simulink model "full_plant20"  (R2021a)
settings: Solver=VariableStepAuto  StartTime=0.0  StopTime=10000  RelTol=1e-3
values from neighbouring files (symbols this model uses):
  alpha_c = 0.00001    (= 1e-05)    [full_plant.m]    (also in full_plant_20.m; policy.m; reactor_core.m)
  alpha_f = -0.00005    (= -5e-05)    [full_plant.m]    (also in full_plant_20.m; policy.m; reactor_core.m)
  beta = p ^ 0.25    (= 0)    [XSteam.m]    (also in XSteam_h_ps.m; full_plant.m = sum(betas); full_plant_20.m = sum(betas); policy.m = sum(betas))
  betas = [0.000215; 0.001424; 0.001274; 0.002568; 0.000748; 0.000273]    [full_plant.m]    (also in full_plant_20.m; policy.m; reactor_core.m)
  err_weights = 0.3    [full_plant_20.m]    (also in sg.m = 0.5)
  eta = 0.85    [PIturing.m]    (also in XSteam.m = h / 3000; XSteam_h_ps.m = h / 3000; full_plant.m = 0.809489; full_plant_20.m = 0.809489)
  eta_all = Pt0 / P_thermal0    [full_plant_20.m]
  ff = 0.98    [full_plant.m]    (also in full_plant_20.m; policy.m; reactor_core.m)
  Gr = 0.0001 * beta    [full_plant_20.m]    (also in reactor_core.m = 0.00001 * beta)
  h_fw = h_sg_out0 - P_thermal0 * 1e3 / num_sg / W_o0    [full_plant.m]    (also in full_plant_20.m; policy.m = h_sg_out0 - P_thermal0 * 1e3 / num_sg / W0; reactor_core.m = h_sg_out0 - P_thermal0 * 1e3 / num_sg / W0; sg.m = h_sg_out0 - P_thermal0 * 1e3 / num_sg / W0)
  J = 8500    [PIturing.m]    (also in full_plant.m; full_plant_20.m; policy.m; reactor_core.m)
  ki_sg = 1.5    [full_plant_20.m]
  kp_sg = 1.6    [full_plant_20.m]
  Lambda = 0.0001    [full_plant.m]    (also in full_plant_20.m; policy.m; reactor_core.m)
  lambdas = [0.0124; 0.0305; 0.1110; 0.3010; 1.1400; 3.0100]    [full_plant.m]    (also in full_plant_20.m; policy.m; reactor_core.m)
  M = M_sg * 2    (= 92.7075812274)    [full_plant.m]    (also in full_plant_20.m; policy.m; reactor_core.m)
  M_sg = P_thermal0 / (T_h0 - T_c0) / num_sg    (= 46.3537906137)    [full_plant.m]    (also in full_plant_20.m; policy.m; reactor_core.m; sg.m)
  mu_c = 70.5    [full_plant.m]    (also in full_plant_20.m; policy.m; reactor_core.m)
  mu_f = 26.3    [full_plant.m]    (also in full_plant_20.m; policy.m; reactor_core.m)
  mu_m = 8.46    [full_plant.m]    (also in full_plant_20.m; policy.m; reactor_core.m; sg.m)
  mu_p = 141.0    (= 141)    [full_plant.m]    (also in full_plant_20.m; policy.m; reactor_core.m; sg.m)
  Ndes = 3600    [PIturing.m]    (also in full_plant.m; full_plant_20.m; policy.m; reactor_core.m)
  num_sg = 2    [full_plant.m]    (also in full_plant_20.m; policy.m; reactor_core.m; sg.m)
  Omega = P_thermal0 * ff / (T_f0 - T_h0)    (= 6.72125630959)    [full_plant.m]    (also in full_plant_20.m; policy.m; reactor_core.m)
  P_sg0 = 6.38    [full_plant.m]    (also in full_plant_20.m; policy.m; reactor_core.m; sg.m)
  P_thermal0 = 2568    [full_plant.m]    (also in full_plant_20.m; policy.m; reactor_core.m; sg.m)
  Pc = 0.008    [PIturing.m]    (also in full_plant.m; full_plant_20.m; policy.m; reactor_core.m)
  Pg0 = 819    [PIturing.m]    (also in full_plant.m = Pt0; full_plant_20.m = Pt0; policy.m = Pt0; reactor_core.m = Pt0)
  SG_gain = 0.002    [full_plant_20.m]
  T_c0 = 290.0    (= 290)    [full_plant.m]    (also in full_plant_20.m; policy.m; reactor_core.m; sg.m)
  T_f0 = 965.28 - 273.15    (= 692.13)    [full_plant.m]    (also in full_plant_20.m; policy.m; reactor_core.m)
  T_h0 = 317.7    [full_plant.m]    (also in full_plant_20.m; policy.m; reactor_core.m; sg.m)
  T_m0 = (T_p0 + T_sg_out0) / 2    [full_plant.m]    (also in full_plant_20.m = (T_c0 + T_sg_out0) / 2; policy.m; reactor_core.m; sg.m)
  T_sg_out0 = XSteam('Tsat_p', P_sg0 * 10)    [full_plant.m]    (also in full_plant_20.m; policy.m; reactor_core.m; sg.m)
  V_f0 = 74.94    [full_plant.m]    (also in full_plant_20.m; policy.m; reactor_core.m; sg.m)
  V_sg = 259.92    [full_plant.m]    (also in full_plant_20.m; policy.m; reactor_core.m; sg.m)
  W_fw0 = 680.4    [full_plant.m]    (also in full_plant_20.m)
  W_steam0 = W_o0 * num_sg    (= 1360.8)    [full_plant_20.m]
  Z1 = P_thermal0 / (T_p0 - T_m0) / num_sg    [full_plant.m]    (also in full_plant_20.m = P_thermal0 / (T_c0 - T_m0) / num_sg; policy.m; reactor_core.m; sg.m)
  Z2 = P_thermal0 / (T_m0 - T_sg_out0) / num_sg    [full_plant.m]    (also in full_plant_20.m; policy.m; reactor_core.m; sg.m)
libraries: simulink x1
settings Model: Creator=xxc90  LastModifiedBy=xxc90

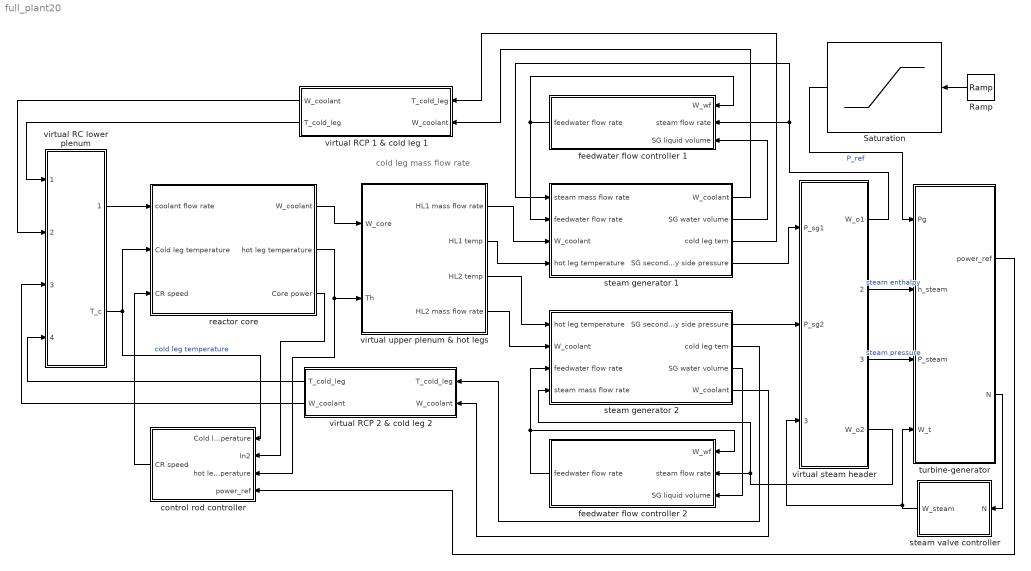
== system full_plant20 ==
  note: cold leg mass flow rate
  Ramp : simulink/Sources/Ramp  slope=-Pg0 * 0.018 / 60  start=10  InitialOutput=Pg0
  Saturation : Saturate  UpperLimit=Pg0  LowerLimit=0.1* Pg0
  control rod controller : Subsystem
  feedwater flow controller 1 : Subsystem
  feedwater flow controller 2 : Subsystem
  reactor core : Subsystem
  steam generator 1 : Subsystem
  steam generator 2 : Subsystem
  steam valve controller : Subsystem
  turbine-generator : Subsystem
  virtual RC lower plenum : MATLAB Function  TreatAsAtomicUnit=on
  virtual RCP 1 & cold leg 1 : MATLAB Function  TreatAsAtomicUnit=on
  virtual RCP 2 & cold leg 2 : MATLAB Function  TreatAsAtomicUnit=on
  virtual steam header : MATLAB Function  TreatAsAtomicUnit=on
  virtual upper plenum & hot legs : Subsystem
  wires:
  virtual RC lower plenum/2(T_c) -> control rod controller/1(Cold leg temperature), reactor core/2(Cold leg temperature)  "cold leg temperature"
  feedwater flow controller 2/1(feedwater flow rate) -> steam generator 2/3(feedwater flow rate), feedwater flow controller 2/1(W_wf)
  steam generator 2/4("W_coolant ") -> virtual RCP 2 & cold leg 2/2("W_coolant ")
  steam generator 1/1("W_coolant ") -> virtual RCP 1 & cold leg 1/2("W_coolant ")
  steam generator 2/2(cold leg tem) -> virtual RCP 2 & cold leg 2/1("T_cold_leg ")
  steam generator 1/3(cold leg tem) -> virtual RCP 1 & cold leg 1/1("T_cold_leg ")
  virtual RCP 2 & cold leg 2/1(T_cold_leg) -> virtual RC lower plenum/4(T_cold_leg2)
  virtual steam header/1(W_o1) -> feedwater flow controller 1/2(steam flow rate), steam generator 1/1(steam mass flow rate)
  feedwater flow controller 1/1(feedwater flow rate) -> steam generator 1/2(feedwater flow rate), feedwater flow controller 1/1(W_wf)
  virtual RCP 2 & cold leg 2/2(W_coolant) -> virtual RC lower plenum/3(W_cold_leg2)
  virtual steam header/4(W_o2) -> steam generator 2/4(steam mass flow rate), feedwater flow controller 2/2(steam flow rate)
  virtual upper plenum & hot legs/2(HL1 temp) -> steam generator 1/4(hot leg temperature)
  virtual upper plenum & hot legs/1(HL1 mass flow rate) -> steam generator 1/3(W_coolant)
  turbine-generator/2(N) -> steam valve controller/1(N)
  turbine-generator/1(power_ref) -> control rod controller/4(power_ref)
  steam valve controller/1(W_steam) -> turbine-generator/4(W_t), virtual steam header/3(W_steam)
  steam generator 1/2(SG water volume) -> feedwater flow controller 1/3(SG liquid volume)
  virtual steam header/3(P_steam) -> turbine-generator/3(P_steam)  "steam pressure"
  reactor core/2(hot leg temperature) -> control rod controller/3(hot leg temperature), virtual upper plenum & hot legs/2(Th)
  steam generator 2/1(SG secondary side pressure) -> virtual steam header/2(P_sg2)
  steam generator 2/3(SG water volume) -> feedwater flow controller 2/3(SG liquid volume)
  virtual RC lower plenum/1(W_core) -> reactor core/1(coolant flow rate)
  reactor core/3(Core power) -> control rod controller/2(In2)
  virtual steam header/2(h_steam) -> turbine-generator/2(h_steam)  "steam enthalpy"
  virtual RCP 1 & cold leg 1/2(T_cold_leg) -> virtual RC lower plenum/1(T_cold_leg1)
  control rod controller/1(CR speed) -> reactor core/3(CR speed)
  steam generator 1/4(SG secondary side pressure) -> virtual steam header/1(P_sg1)
  virtual upper plenum & hot legs/3(HL2 temp) -> steam generator 2/1(hot leg temperature)
  virtual upper plenum & hot legs/4(HL2 mass flow rate) -> steam generator 2/2(W_coolant)
  reactor core/1("W_coolant ") -> virtual upper plenum & hot legs/1(W_core)
  virtual RCP 1 & cold leg 1/1(W_coolant) -> virtual RC lower plenum/2(W_cold_leg1)
  Ramp/1 -> Saturation/1
  Saturation/1 -> turbine-generator/1(Pg)  "P_ref"

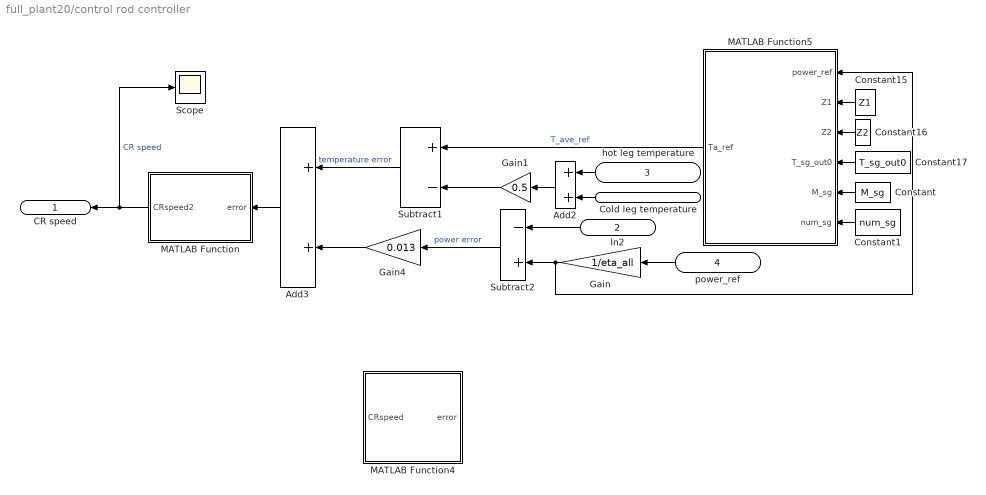
== system full_plant20/control rod controller ==
  Cold leg temperature : Inport
  In2 : Inport  Port=2
  hot leg temperature : Inport  Port=3
  power_ref : Inport  Port=4
  Add2 : Sum
  Add3 : Sum
  Constant : Constant  Value=M_sg
  Constant1 : Constant  Value=num_sg
  Constant15 : Constant  Value=Z1
  Constant16 : Constant  Value=Z2
  Constant17 : Constant  Value=T_sg_out0
  Gain : Gain  Gain=1/eta_all
  Gain1 : Gain  Gain=0.5
  Gain4 : Gain  Gain=0.013
  MATLAB Function : MATLAB Function  TreatAsAtomicUnit=on
  MATLAB Function4 : MATLAB Function  TreatAsAtomicUnit=on
  MATLAB Function5 : MATLAB Function  TreatAsAtomicUnit=on
  Scope : Scope
  Subtract1 : Sum  Inputs=+-
  Subtract2 : Sum  Inputs=-+
  CR speed : Outport
  wires:
  In2/1 -> Subtract2/1
  hot leg temperature/1 -> Add2/1
  Add2/1 -> Gain1/1
  Cold leg temperature/1 -> Add2/2
  MATLAB Function/1(CRspeed2) -> Scope/1, CR speed/1  "CR speed"
  Subtract2/1 -> Gain4/1  "power error"
  Constant15/1 -> MATLAB Function5/2(Z1)
  Subtract1/1 -> Add3/1  "temperature error"
  Gain4/1 -> Add3/2
  Constant17/1 -> MATLAB Function5/4(T_sg_out0)
  MATLAB Function5/1(Ta_ref) -> Subtract1/1  "T_ave_ref"
  Constant16/1 -> MATLAB Function5/3(Z2)
  power_ref/1 -> Gain/1
  Gain/1 -> MATLAB Function5/1(power_ref), Subtract2/2
  Constant/1 -> MATLAB Function5/5(M_sg)
  Constant1/1 -> MATLAB Function5/6(num_sg)
  Gain1/1 -> Subtract1/2
  Add3/1 -> MATLAB Function/1(error)

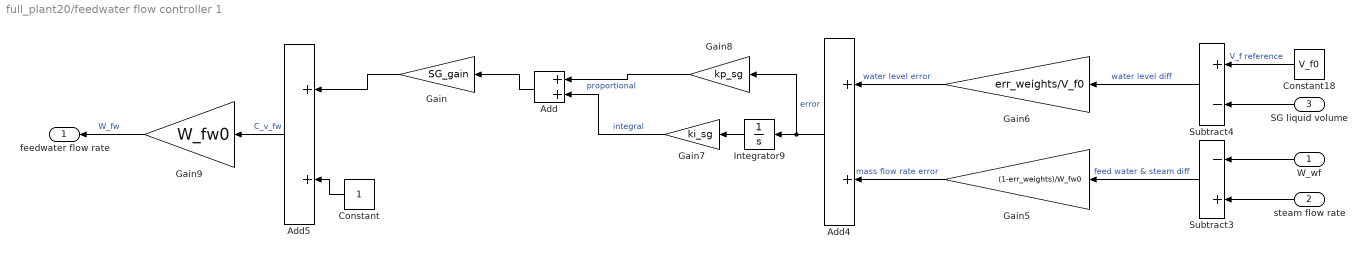
== system full_plant20/feedwater flow controller 1 ==
  W_wf : Inport
  steam flow rate : Inport  Port=2
  SG liquid volume : Inport  Port=3
  Add : Sum
  Add4 : Sum
  Add5 : Sum
  Constant : Constant
  Constant18 : Constant  Value=V_f0
  Gain : Gain  Gain=SG_gain
  Gain5 : Gain  Gain=(1-err_weights)/W_fw0
  Gain6 : Gain  Gain=err_weights/V_f0
  Gain7 : Gain  Gain=ki_sg
  Gain8 : Gain  Gain=kp_sg
  Gain9 : Gain  Gain=W_fw0
  Integrator9 : Integrator
  Subtract3 : Sum  Inputs=-+
  Subtract4 : Sum  Inputs=+-
  feedwater flow rate : Outport
  wires:
  steam flow rate/1 -> Subtract3/2
  Gain5/1 -> Add4/2  "mass flow rate error"
  Add5/1 -> Gain9/1  "C_v_fw"
  Constant18/1 -> Subtract4/1  "V_f reference"
  Subtract4/1 -> Gain6/1  "water level diff"
  Gain9/1 -> feedwater flow rate/1  "W_fw"
  Add4/1 -> Gain8/1, Integrator9/1  "error"
  Gain6/1 -> Add4/1  "water level error"
  SG liquid volume/1 -> Subtract4/2
  W_wf/1 -> Subtract3/1
  Integrator9/1 -> Gain7/1
  Subtract3/1 -> Gain5/1  "feed water & steam diff"
  Constant/1 -> Add5/2
  Gain/1 -> Add5/1
  Gain8/1 -> Add/1  "proportional"
  Gain7/1 -> Add/2  "integral"
  Add/1 -> Gain/1

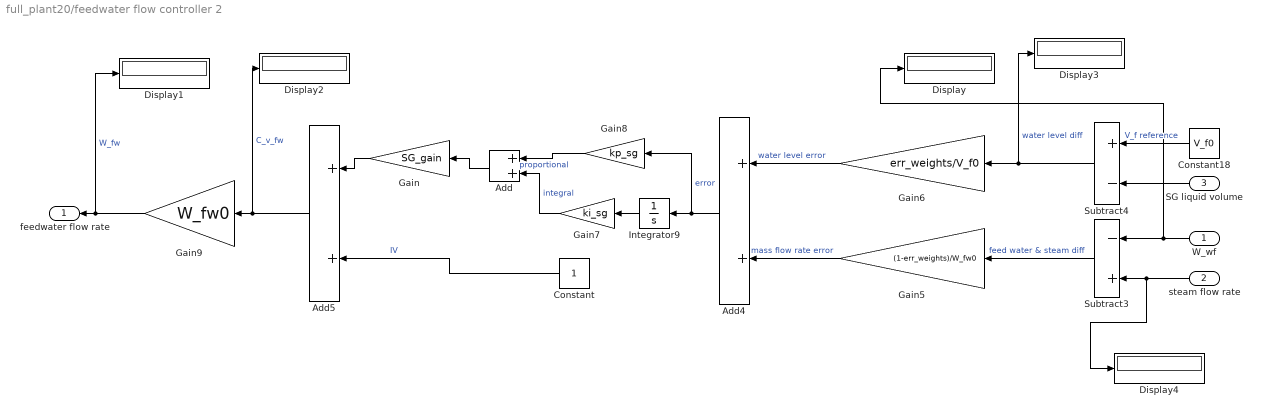
== system full_plant20/feedwater flow controller 2 ==
  W_wf : Inport
  steam flow rate : Inport  Port=2
  SG liquid volume : Inport  Port=3
  Add : Sum
  Add4 : Sum
  Add5 : Sum
  Constant : Constant
  Constant18 : Constant  Value=V_f0
  Display{,1..4} (5 alike) : Display
  Gain : Gain  Gain=SG_gain
  Gain5 : Gain  Gain=(1-err_weights)/W_fw0
  Gain6 : Gain  Gain=err_weights/V_f0
  Gain7 : Gain  Gain=ki_sg
  Gain8 : Gain  Gain=kp_sg
  Gain9 : Gain  Gain=W_fw0
  Integrator9 : Integrator
  Subtract3 : Sum  Inputs=-+
  Subtract4 : Sum  Inputs=+-
  feedwater flow rate : Outport
  wires:
  Gain5/1 -> Add4/2  "mass flow rate error"
  Add5/1 -> Display2/1, Gain9/1  "C_v_fw"
  Constant18/1 -> Subtract4/1  "V_f reference"
  Subtract4/1 -> Display3/1, Gain6/1  "water level diff"
  Gain9/1 -> Display1/1, feedwater flow rate/1  "W_fw"
  Add4/1 -> Gain8/1, Integrator9/1  "error"
  Gain6/1 -> Add4/1  "water level error"
  SG liquid volume/1 -> Subtract4/2
  W_wf/1 -> Display/1, Subtract3/1
  Integrator9/1 -> Gain7/1
  Subtract3/1 -> Gain5/1  "feed water & steam diff"
  Constant/1 -> Add5/2  "IV"
  steam flow rate/1 -> Display4/1, Subtract3/2
  Gain8/1 -> Add/1  "proportional"
  Gain7/1 -> Add/2  "integral"
  Add/1 -> Gain/1
  Gain/1 -> Add5/1

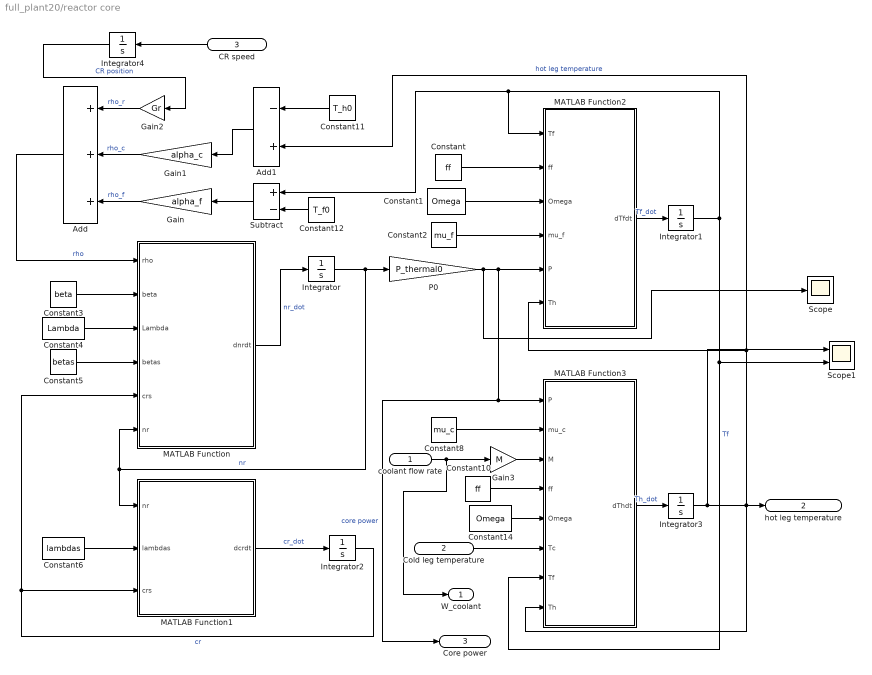
== system full_plant20/reactor core ==
  coolant flow rate : Inport
  Cold leg temperature : Inport  Port=2
  CR speed : Inport  Port=3
  Add : Sum  Inputs=+++
  Add1 : Sum  Inputs=-+
  Constant : Constant  Value=ff
  Constant1 : Constant  Value=Omega
  Constant10 : Constant  Value=ff
  Constant11 : Constant  Value=T_h0
  Constant12 : Constant  Value=T_f0
  Constant14 : Constant  Value=Omega
  Constant2 : Constant  Value=mu_f
  Constant3 : Constant  Value=beta
  Constant4 : Constant  Value=Lambda
  Constant5 : Constant  Value=betas
  Constant6 : Constant  Value=lambdas
  Constant8 : Constant  Value=mu_c
  Gain : Gain  Gain=alpha_f
  Gain1 : Gain  Gain=alpha_c
  Gain2 : Gain  Gain=Gr
  Gain3 : Gain  Gain=M
  Integrator : Integrator  InitialCondition=1
  Integrator1 : Integrator  InitialCondition=T_f0
  Integrator2 : Integrator  InitialCondition=[1;1;1;1;1;1]
  Integrator3 : Integrator  InitialCondition=T_h0
  Integrator4 : Integrator
  MATLAB Function : MATLAB Function  TreatAsAtomicUnit=on
  MATLAB Function1 : MATLAB Function  TreatAsAtomicUnit=on
  MATLAB Function2 : MATLAB Function  TreatAsAtomicUnit=on
  MATLAB Function3 : MATLAB Function  TreatAsAtomicUnit=on
  P0 : Gain  Gain=P_thermal0
  Scope : Scope
  Scope1 : Scope  NumInputPorts=2
  Subtract : Sum  Inputs=+-
  "W_coolant " : Outport
  hot leg temperature : Outport  Port=2
  Core power : Outport  Port=3
  wires:
  MATLAB Function3/1(dThdt) -> Integrator3/1  "Th_dot"
  Constant14/1 -> MATLAB Function3/5(Omega)
  Constant/1 -> MATLAB Function2/2(ff)
  Add/1 -> MATLAB Function/1(rho)  "rho"
  Integrator4/1 -> Gain2/1  "CR position"
  Add1/1 -> Gain1/1
  Gain/1 -> Add/3  "rho_f"
  Integrator2/1 -> MATLAB Function/5(crs), MATLAB Function1/3(crs)  "cr"
  Constant11/1 -> Add1/1
  MATLAB Function/1(dnrdt) -> Integrator/1  "nr_dot"
  MATLAB Function1/1(dcrdt) -> Integrator2/1  "cr_dot"
  Cold leg temperature/1 -> MATLAB Function3/6(Tc)
  Constant1/1 -> MATLAB Function2/3(Omega)
  Gain2/1 -> Add/1  "rho_r"
  CR speed/1 -> Integrator4/1
  Constant3/1 -> MATLAB Function/2(beta)
  Integrator1/1 -> MATLAB Function2/1(Tf), Subtract/1, Scope1/2, MATLAB Function3/7(Tf)  "Tf"
  Integrator3/1 -> Scope1/1, hot leg temperature/1, MATLAB Function3/8(Th), Add1/2, MATLAB Function2/6(Th)  "hot leg temperature"
  Constant4/1 -> MATLAB Function/3(Lambda)
  Gain1/1 -> Add/2  "rho_c"
  P0/1 -> Scope/1, Core power/1, MATLAB Function3/1(P), MATLAB Function2/5(P)  "core power"
  Constant8/1 -> MATLAB Function3/2(mu_c)
  Constant10/1 -> MATLAB Function3/4(ff)
  Constant2/1 -> MATLAB Function2/4(mu_f)
  Integrator/1 -> P0/1, MATLAB Function/6(nr), MATLAB Function1/1(nr)  "nr"
  MATLAB Function2/1(dTfdt) -> Integrator1/1  "Tf_dot"
  Constant5/1 -> MATLAB Function/4(betas)
  Constant6/1 -> MATLAB Function1/2(lambdas)
  Constant12/1 -> Subtract/2
  Gain3/1 -> MATLAB Function3/3(M)
  Subtract/1 -> Gain/1
  coolant flow rate/1 -> Gain3/1, "W_coolant "/1

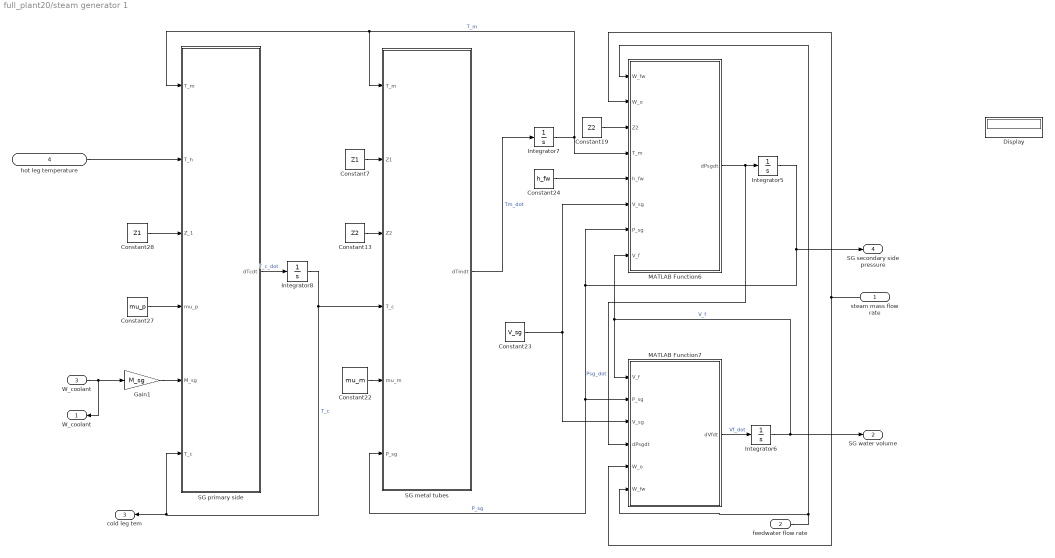
== system full_plant20/steam generator 1 ==
  steam mass flow rate : Inport
  feedwater flow rate : Inport  Port=2
  W_coolant : Inport  Port=3
  hot leg temperature : Inport  Port=4
  Constant13 : Constant  Value=Z2
  Constant19 : Constant  Value=Z2
  Constant22 : Constant  Value=mu_m
  Constant23 : Constant  Value=V_sg
  Constant24 : Constant  Value=h_fw
  Constant27 : Constant  Value=mu_p
  Constant28 : Constant  Value=Z1
  Constant7 : Constant  Value=Z1
  Display : Display
  Gain1 : Gain  Gain=M_sg
  Integrator5 : Integrator  InitialCondition=P_sg0
  Integrator6 : Integrator  InitialCondition=V_f0
  Integrator7 : Integrator  InitialCondition=T_m0
  Integrator8 : Integrator  InitialCondition=T_c0
  MATLAB Function6 : MATLAB Function  TreatAsAtomicUnit=on
  MATLAB Function7 : MATLAB Function  TreatAsAtomicUnit=on
  SG metal tubes : MATLAB Function  TreatAsAtomicUnit=on
  SG primary side : MATLAB Function  TreatAsAtomicUnit=on
  "W_coolant " : Outport
  SG water volume : Outport  Port=2
  cold leg tem : Outport  Port=3
  SG secondary side pressure : Outport  Port=4
  wires:
  Constant19/1 -> MATLAB Function6/3(Z2)
  feedwater flow rate/1 -> MATLAB Function7/6(W_fw), MATLAB Function6/1(W_fw)
  SG primary side/1(dTcdt) -> Integrator8/1  "T_c_dot"
  Constant7/1 -> SG metal tubes/2(Z1)
  Integrator8/1 -> SG metal tubes/4(T_c), cold leg tem/1, SG primary side/6(T_c)  "T_c"
  Integrator5/1 -> MATLAB Function7/2(P_sg), SG metal tubes/6(P_sg), MATLAB Function6/7(P_sg), SG secondary side pressure/1  "P_sg"
  Constant24/1 -> MATLAB Function6/5(h_fw)
  SG metal tubes/1(dTmdt) -> Integrator7/1  "Tm_dot"
  hot leg temperature/1 -> SG primary side/2(T_h)
  Constant23/1 -> MATLAB Function7/3(V_sg), MATLAB Function6/6(V_sg)
  Integrator6/1 -> SG water volume/1, MATLAB Function7/1(V_f), MATLAB Function6/8(V_f)  "V_f"
  steam mass flow rate/1 -> MATLAB Function7/5(W_o), MATLAB Function6/2(W_o)
  MATLAB Function6/1(dPsgdt) -> Integrator5/1, MATLAB Function7/4(dPsgdt)  "Psg_dot"
  Constant22/1 -> SG metal tubes/5(mu_m)
  Constant13/1 -> SG metal tubes/3(Z2)
  Constant28/1 -> SG primary side/3(Z_1)
  Gain1/1 -> SG primary side/5(M_sg)
  MATLAB Function7/1(dVfdt) -> Integrator6/1  "Vf_dot"
  Integrator7/1 -> SG primary side/1(T_m), SG metal tubes/1(T_m), MATLAB Function6/4(T_m)  "T_m"
  Constant27/1 -> SG primary side/4(mu_p)
  W_coolant/1 -> "W_coolant "/1, Gain1/1

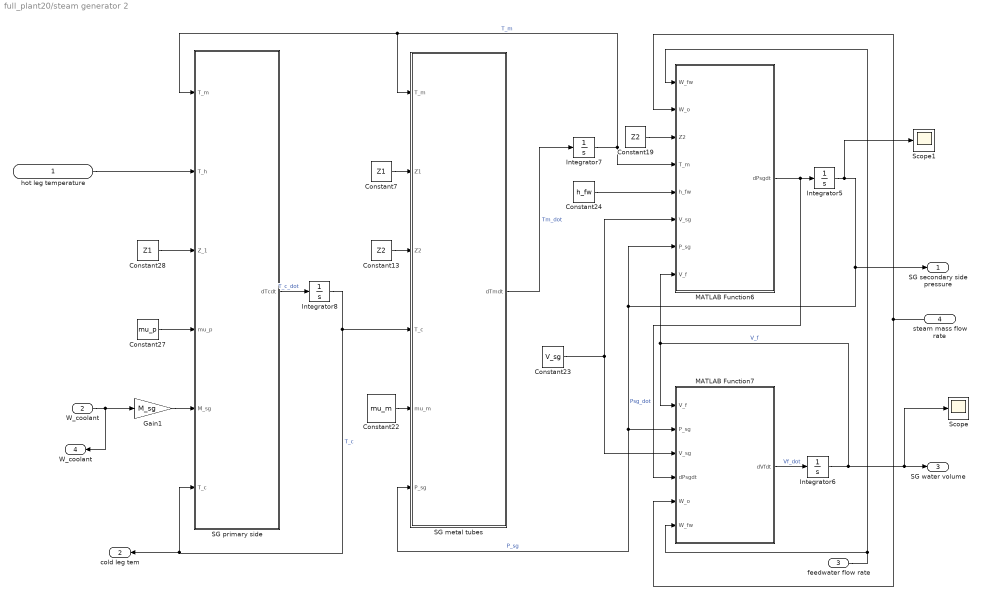
== system full_plant20/steam generator 2 ==
  hot leg temperature : Inport
  W_coolant : Inport  Port=2
  feedwater flow rate : Inport  Port=3
  steam mass flow rate : Inport  Port=4
  Constant13 : Constant  Value=Z2
  Constant19 : Constant  Value=Z2
  Constant22 : Constant  Value=mu_m
  Constant23 : Constant  Value=V_sg
  Constant24 : Constant  Value=h_fw
  Constant27 : Constant  Value=mu_p
  Constant28 : Constant  Value=Z1
  Constant7 : Constant  Value=Z1
  Gain1 : Gain  Gain=M_sg
  Integrator5 : Integrator  InitialCondition=P_sg0
  Integrator6 : Integrator  InitialCondition=V_f0
  Integrator7 : Integrator  InitialCondition=T_m0
  Integrator8 : Integrator  InitialCondition=T_c0
  MATLAB Function6 : MATLAB Function  TreatAsAtomicUnit=on
  MATLAB Function7 : MATLAB Function  TreatAsAtomicUnit=on
  SG metal tubes : MATLAB Function  TreatAsAtomicUnit=on
  SG primary side : MATLAB Function  TreatAsAtomicUnit=on
  Scope : Scope
  Scope1 : Scope
  SG secondary side pressure : Outport
  cold leg tem : Outport  Port=2
  SG water volume : Outport  Port=3
  "W_coolant " : Outport  Port=4
  wires:
  Constant19/1 -> MATLAB Function6/3(Z2)
  feedwater flow rate/1 -> MATLAB Function7/6(W_fw), MATLAB Function6/1(W_fw)
  SG primary side/1(dTcdt) -> Integrator8/1  "T_c_dot"
  Constant7/1 -> SG metal tubes/2(Z1)
  Integrator8/1 -> SG metal tubes/4(T_c), cold leg tem/1, SG primary side/6(T_c)  "T_c"
  Integrator5/1 -> Scope1/1, MATLAB Function7/2(P_sg), SG metal tubes/6(P_sg), MATLAB Function6/7(P_sg), SG secondary side pressure/1  "P_sg"
  Constant24/1 -> MATLAB Function6/5(h_fw)
  SG metal tubes/1(dTmdt) -> Integrator7/1  "Tm_dot"
  hot leg temperature/1 -> SG primary side/2(T_h)
  Constant23/1 -> MATLAB Function7/3(V_sg), MATLAB Function6/6(V_sg)
  Integrator6/1 -> Scope/1, SG water volume/1, MATLAB Function7/1(V_f), MATLAB Function6/8(V_f)  "V_f"
  steam mass flow rate/1 -> MATLAB Function7/5(W_o), MATLAB Function6/2(W_o)
  MATLAB Function6/1(dPsgdt) -> Integrator5/1, MATLAB Function7/4(dPsgdt)  "Psg_dot"
  Constant22/1 -> SG metal tubes/5(mu_m)
  Constant13/1 -> SG metal tubes/3(Z2)
  Constant28/1 -> SG primary side/3(Z_1)
  Gain1/1 -> SG primary side/5(M_sg)
  MATLAB Function7/1(dVfdt) -> Integrator6/1  "Vf_dot"
  Integrator7/1 -> SG primary side/1(T_m), SG metal tubes/1(T_m), MATLAB Function6/4(T_m)  "T_m"
  Constant27/1 -> SG primary side/4(mu_p)
  W_coolant/1 -> "W_coolant "/1, Gain1/1

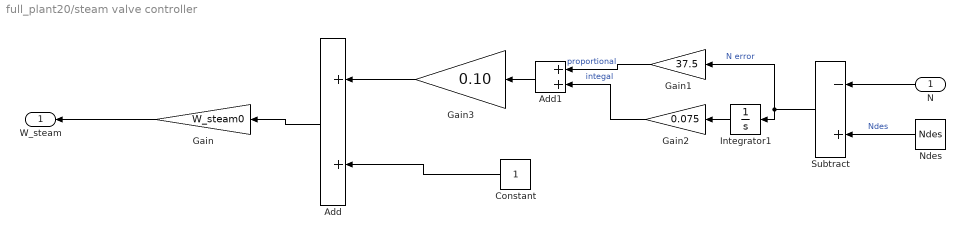
== system full_plant20/steam valve controller ==
  N : Inport
  Add : Sum
  Add1 : Sum
  Constant : Constant
  Gain : Gain  Gain=W_steam0
  Gain1 : Gain  Gain=37.5
  Gain2 : Gain  Gain=0.075
  Gain3 : Gain  Gain=0.10
  Integrator1 : Integrator
  Ndes : Constant  Value=Ndes
  Subtract : Sum  Inputs=-+
  W_steam : Outport
  wires:
  Gain2/1 -> Add1/2  "integal"
  Ndes/1 -> Subtract/2  "Ndes"
  N/1 -> Subtract/1
  Gain/1 -> W_steam/1
  Integrator1/1 -> Gain2/1
  Subtract/1 -> Gain1/1, Integrator1/1  "N error"
  Add/1 -> Gain/1
  Gain1/1 -> Add1/1  "proportional"
  Constant/1 -> Add/2
  Add1/1 -> Gain3/1
  Gain3/1 -> Add/1

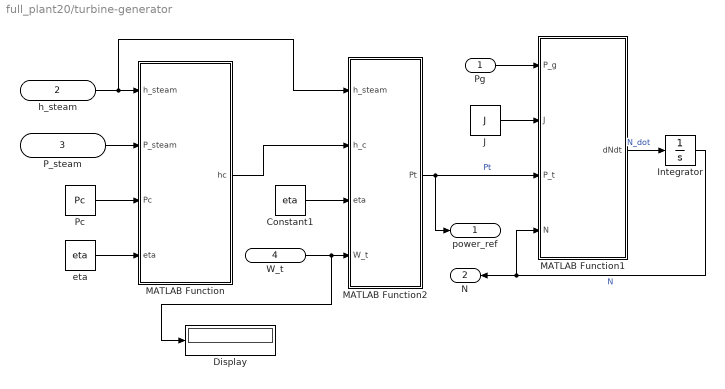
== system full_plant20/turbine-generator ==
  Pg : Inport
  h_steam : Inport  Port=2
  P_steam : Inport  Port=3
  W_t : Inport  Port=4
  Constant1 : Constant  Value=eta
  Display : Display
  Integrator : Integrator  InitialCondition=3600
  J : Constant  Value=J
  MATLAB Function : MATLAB Function  TreatAsAtomicUnit=on
  MATLAB Function1 : MATLAB Function  TreatAsAtomicUnit=on
  MATLAB Function2 : MATLAB Function  TreatAsAtomicUnit=on
  Pc : Constant  Value=Pc
  eta : Constant  Value=eta
  power_ref : Outport
  N : Outport  Port=2
  wires:
  W_t/1 -> Display/1, MATLAB Function2/4(W_t)
  P_steam/1 -> MATLAB Function/2(P_steam)
  Pc/1 -> MATLAB Function/3(Pc)
  MATLAB Function1/1(dNdt) -> Integrator/1  "N_dot"
  eta/1 -> MATLAB Function/4(eta)
  Pg/1 -> MATLAB Function1/1(P_g)
  Constant1/1 -> MATLAB Function2/3(eta)
  Integrator/1 -> MATLAB Function1/4(N), N/1  "N"
  h_steam/1 -> MATLAB Function2/1(h_steam), MATLAB Function/1(h_steam)
  J/1 -> MATLAB Function1/2(J)
  MATLAB Function/1(hc) -> MATLAB Function2/2(h_c)
  MATLAB Function2/1(Pt) -> MATLAB Function1/3(P_t), power_ref/1  "Pt"

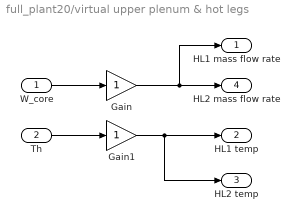
== system full_plant20/virtual upper plenum & hot legs ==
  W_core : Inport
  Th : Inport  Port=2
  Gain : Gain
  Gain1 : Gain
  HL1 mass flow rate : Outport
  HL1 temp : Outport  Port=2
  HL2 temp : Outport  Port=3
  HL2 mass flow rate : Outport  Port=4
  wires:
  Th/1 -> Gain1/1
  Gain/1 -> HL1 mass flow rate/1, HL2 mass flow rate/1
  W_core/1 -> Gain/1
  Gain1/1 -> HL2 temp/1, HL1 temp/1

== matlab function full_plant20/steam generator 1/SG primary side ==
  data: T_m input; T_h input; Z_1 input; mu_p input; M_sg input; dTcdt output; T_c input
function dTcdt = dTcdt(T_m, T_h, Z_1, mu_p, M_sg, T_c)
    dTcdt = (M_sg * (T_h - T_c) - Z_1 * (T_c - T_m)) / mu_p
end

== matlab function full_plant20/steam generator 1/SG metal tubes ==
  data: T_m input; dTmdt output; Z1 input; Z2 input; T_c input; mu_m input; P_sg input
function dTmdt = dTmdt(T_m, Z1, Z2, T_c, mu_m, P_sg)
    T_s = XSteam('Tsat_p', P_sg*10);
    dTmdt = (Z1 * (T_c - T_m) - Z2*(T_m - T_s)) / mu_m
end

== matlab function full_plant20/steam generator 2/MATLAB Function6 ==
  data: W_fw input; dPsgdt output; W_o input; Z2 input; T_m input; h_fw input; V_sg input; P_sg input; V_f input
function dPsgdt= dPsgdt(W_fw, W_o, Z2, T_m, h_fw, V_sg, P_sg, V_f)
    T_s = XSteam('Tsat_p', P_sg*10);
    rho_g = XSteam('rhoV_p', P_sg*10);
    u_g = XSteam('uV_p', P_sg*10);
    h_g = XSteam('hV_p', P_sg*10)
    rho_f = XSteam('rhoL_p', P_sg*10);
    u_f = XSteam('uL_p', P_sg*10);
    dP = 0.01;
    dufdP = (XSteam('uL_p', P_sg*10+ dP) - XSteam('uL_p', P_sg*10)) / dP;
    dugdP = (XSteam('uV_p', P_sg*10+ dP) - XSteam('uV_p', P_sg*10)) / dP;
    drhofdP = (XSteam('rhoL_p', P_sg*10+ dP) - XSteam('rhoL_p', P_sg*10)) / dP;
    drhogdP = (XSteam('rhoV_p', P_sg*10+ dP) - XSteam('rhoV_p', P_sg*10)) / dP;
    dPsgdt_num = W_fw * h_fw - W_o * h_g + Z2 * (T_m - T_s) * 1000 + (rho_g*u_g - rho_f*u_f)/(rho_f-rho_g)*(W_fw - W_o);
    dPsgdt_den = rho_f * V_f * dufdP + (V_sg - V_f) * u_g * drhogdP + rho_g * (V_sg - V_f) * dugdP + (V_sg - V_f) * (rho_g*u_g - rho_f*u_f)/(rho_f-rho_g) * drhogdP ;
    dPsgdt = dPsgdt_num / dPsgdt_den;
end

== matlab function full_plant20/steam generator 2/MATLAB Function7 ==
  data: V_f input; P_sg input; V_sg input; dPsgdt input; W_o input; W_fw input; dVfdt output
function dVfdt = dVfdt(V_f, P_sg, V_sg, dPsgdt, W_o, W_fw)
    rho_f = XSteam('rhoL_p', P_sg*10);
    rho_g = XSteam('rhoV_p', P_sg*10);
    dP = 0.01;
    drhogdP = (XSteam('rhoV_p', P_sg*10+ dP) - XSteam('rhoV_p', P_sg*10)) / dP;
    dVfdt = (W_fw - W_o - (V_sg - V_f)* drhogdP * dPsgdt) / (rho_f - rho_g);
end

== matlab function full_plant20/reactor core/MATLAB Function1 ==
  data: nr input; lambdas input; dcrdt output; crs input
function dcrdt = dcrdt(nr, lambdas, crs)
    dcrdt = lambdas * nr - lambdas .* crs;
end

== matlab function full_plant20/steam generator 2/SG metal tubes ==
  data: T_m input; dTmdt output; Z1 input; Z2 input; T_c input; mu_m input; P_sg input
function dTmdt = dTmdt(T_m, Z1, Z2, T_c, mu_m, P_sg)
    T_s = XSteam('Tsat_p', P_sg*10);
    dTmdt = (Z1 * (T_c - T_m) - Z2*(T_m - T_s)) / mu_m
end

== matlab function full_plant20/steam generator 2/SG primary side ==
  data: T_m input; T_h input; Z_1 input; mu_p input; M_sg input; dTcdt output; T_c input
function dTcdt = dTcdt(T_m, T_h, Z_1, mu_p, M_sg, T_c)
    dTcdt = (M_sg * (T_h - T_c) - Z_1 * (T_c - T_m)) / mu_p
end

== matlab function full_plant20/turbine-generator/MATLAB Function ==
  data: h_steam input; P_steam input; Pc input; hc output; eta input
function hc = hc(h_steam,  P_steam, Pc, eta)
    hc = 0;
    fun = 'h_ps';
    s_steam = XSteam('sV_p', P_steam * 10)
    hc = h_steam - eta * (h_steam - XSteam_h_ps(fun, Pc*10, s_steam));
end

== matlab function full_plant20/turbine-generator/MATLAB Function1 ==
  data: P_g input; J input; dNdt output; P_t input; N input
function dNdt = dNdt(P_g, J, P_t, N)
    dNdt = (60 / (2*pi))^2 * (P_t - P_g) / (J*N);
end

== matlab function full_plant20/turbine-generator/MATLAB Function2 ==
  data: h_steam input; Pt output; h_c input; eta input; W_t input
function Pt = Pt(h_steam, h_c, eta, W_t)
    Pt = (h_steam - h_c) * W_t * eta / 1000;
end

== matlab function full_plant20/virtual RCP 1 & cold leg 1 ==
  data: T_cold_leg input; W_coolant output; T_cold_leg output; W_coolant input
function [W_coolant, T_cold_leg] = fcn(T_cold_leg, W_coolant)
    W_coolant = 1
end

== matlab function full_plant20/virtual steam header ==
  data: W_o1 output; P_sg1 input; P_sg2 input; h_steam output; P_steam output; W_steam input; W_o2 output
function [W_o1, h_steam, P_steam, W_o2] = fcn(P_sg1, P_sg2, W_steam)
    h_steam = XSteam('hV_p', P_sg1 * 10);
    P_steam = P_sg2;
    W_o1 = W_steam / 2;
    W_o2 = W_steam / 2;
end

== matlab function full_plant20/virtual RC lower plenum ==
  data: W_core output; T_c output; T_cold_leg1 input; W_cold_leg1 input; W_cold_leg2 input; T_cold_leg2 input
function [W_core, T_c]  = fcn(T_cold_leg1, W_cold_leg1, W_cold_leg2, T_cold_leg2)
    W_core = (W_cold_leg1 + W_cold_leg2) / 2;
    T_c = T_cold_leg1;
end

== matlab function full_plant20/reactor core/MATLAB Function ==
  data: rho input; dnrdt output size=1; beta input; Lambda input; betas input; crs input; nr input
function dnrdt= dnrdt(rho, beta, Lambda, betas, crs, nr)
    dnrdt = (rho - beta) / Lambda * nr + betas' / Lambda * crs;
end

== matlab function full_plant20/virtual RCP 2 & cold leg 2 ==
  data: T_cold_leg output; T_cold_leg input; W_coolant output; W_coolant input
function [T_cold_leg, W_coolant] = fcn(T_cold_leg, W_coolant)
    W_coolant = 1
end

== matlab function full_plant20/control rod controller/MATLAB Function ==
  data: error input; CRspeed2 output
function CRspeed2 = CRspeed2(error)
    error_F = error * 9 / 5;
    if error_F < -6
        CRspeed2 = -72
    elseif (error_F >= -6) && (error_F <= 6)
        CRspeed2 = 12 * error_F
    else CRspeed2 = 72

    end
end

== matlab function full_plant20/reactor core/MATLAB Function2 ==
  data: Tf input; ff input; Omega input; mu_f input; P input; Th input; dTfdt output
function dTfdt = dTfdt(Tf, ff, Omega, mu_f, P, Th)
    dTfdt = (ff * P - Omega *(Tf - Th)) / mu_f
end

== matlab function full_plant20/reactor core/MATLAB Function3 ==
  data: P input; dThdt output; mu_c input; M input; ff input; Omega input; Tc input; Tf input; Th input
function dThdt = dThdt(P, mu_c, M, ff, Omega, Tc, Tf, Th)
    dThdt = ((1-ff)*P + Omega*(Tf-Th) - M*(Th - Tc)) / mu_c
end

== matlab function full_plant20/control rod controller/MATLAB Function4 ==
  data: error input; CRspeed output
function CRspeed = CRspeed(error)
    error_F = error * 9 / 5;
    if error_F < -5
        CRspeed = -72;
    elseif (error_F >= -5) && (error_F<=-3)
        CRspeed = 88 + 32 * error_F;
    elseif (error_F > -3) && (error_F<-1)
        CRspeed = -8;
    elseif (error_F >= -1) && (error_F<= 1)
        CRspeed = 0;
    elseif (error_F > 1) && (error_F<3)
        CRspeed = 8;
    elseif (error_F >= 3) && (error_F<=5)
        CRspeed = -88 + 32 * error_F;
    else
        CRspeed = 72
end

== matlab function full_plant20/control rod controller/MATLAB Function5 ==
  data: power_ref input; Ta_ref output; Z1 input; Z2 input; T_sg_out0 input; M_sg input; num_sg input
function Ta_ref = Ta_ref(power_ref, Z1, Z2, T_sg_out0, M_sg, num_sg)
    power_ref = power_ref / num_sg;
    T_c_h_diff_policy = power_ref / M_sg;
    T_c_policy = power_ref / Z1 + power_ref / Z2 + T_sg_out0;
    T_h_policy = T_c_policy + T_c_h_diff_policy; 
    Ta_ref = (T_c_policy + T_h_policy) / 2;
end

== matlab function full_plant20/steam generator 1/MATLAB Function6 ==
  data: W_fw input; dPsgdt output; W_o input; Z2 input; T_m input; h_fw input; V_sg input; P_sg input; V_f input
function dPsgdt= dPsgdt(W_fw, W_o, Z2, T_m, h_fw, V_sg, P_sg, V_f)
    T_s = XSteam('Tsat_p', P_sg*10);
    rho_g = XSteam('rhoV_p', P_sg*10);
    u_g = XSteam('uV_p', P_sg*10);
    h_g = XSteam('hV_p', P_sg*10)
    rho_f = XSteam('rhoL_p', P_sg*10);
    u_f = XSteam('uL_p', P_sg*10);
    dP = 0.01;
    dufdP = (XSteam('uL_p', P_sg*10+ dP) - XSteam('uL_p', P_sg*10)) / dP;
    dugdP = (XSteam('uV_p', P_sg*10+ dP) - XSteam('uV_p', P_sg*10)) / dP;
    drhofdP = (XSteam('rhoL_p', P_sg*10+ dP) - XSteam('rhoL_p', P_sg*10)) / dP;
    drhogdP = (XSteam('rhoV_p', P_sg*10+ dP) - XSteam('rhoV_p', P_sg*10)) / dP;
    dPsgdt_num = W_fw * h_fw - W_o * h_g + Z2 * (T_m - T_s) * 1000 + (rho_g*u_g - rho_f*u_f)/(rho_f-rho_g)*(W_fw - W_o);
    dPsgdt_den = rho_f * V_f * dufdP + (V_sg - V_f) * u_g * drhogdP + rho_g * (V_sg - V_f) * dugdP + (V_sg - V_f) * (rho_g*u_g - rho_f*u_f)/(rho_f-rho_g) * drhogdP ;
    dPsgdt = dPsgdt_num / dPsgdt_den;
end

== matlab function full_plant20/steam generator 1/MATLAB Function7 ==
  data: V_f input; P_sg input; V_sg input; dPsgdt input; W_o input; W_fw input; dVfdt output
function dVfdt = dVfdt(V_f, P_sg, V_sg, dPsgdt, W_o, W_fw)
    rho_f = XSteam('rhoL_p', P_sg*10);
    rho_g = XSteam('rhoV_p', P_sg*10);
    dP = 0.01;
    drhogdP = (XSteam('rhoV_p', P_sg*10+ dP) - XSteam('rhoV_p', P_sg*10)) / dP;
    dVfdt = (W_fw - W_o - (V_sg - V_f)* drhogdP * dPsgdt) / (rho_f - rho_g);
end
